simulink model "eq_2khz"  (R2023a)
settings: Solver=VariableStepAuto  StartTime=0.0  StopTime=5.0  RelTol=1e-3
libraries: spspowerguiLib x1
settings Model: Creator=若陈不生病  LastModifiedBy=86198

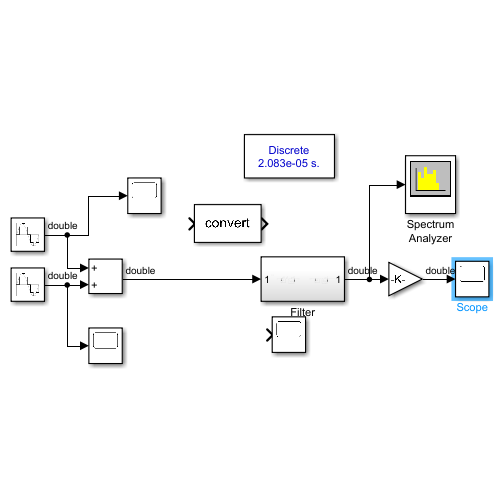
[thumbnail: Simulink's stored preview of the top-level diagram]
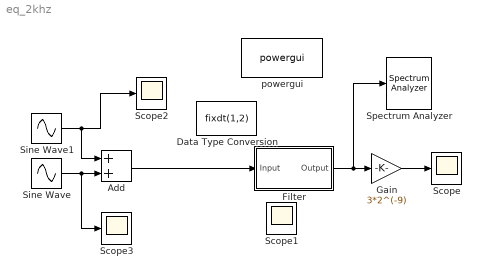
== system eq_2khz ==
  Add : Sum
  Data Type Conversion : DataTypeConversion  OutMin=[-1.1/1.5]  OutMax=[1.1/1.5]  OutDataTypeStr=fixdt(1,2)  SaturateOnIntegerOverflow=off  RndMeth=Floor
  Filter : Subsystem  Tag=FilterWizardSubSystem
      settings: ErrorFcn=dspFilterRealizedInBasicElemsAlgLoopErrFcnCallback
  Gain : Gain  Gain=3*2^(-9)
  Scope{,1..3} (4 alike) : Scope
  Sine Wave : Sin  Frequency=2*pi*200  SampleTime=1/48000
  Sine Wave1 : Sin  Frequency=2*pi*2000  SampleTime=1/48000
  Spectrum Analyzer : SpectrumAnalyzer  WindowPosition=[320.000000,230.000000,800.000000,500.000000,]  Visible=on  ScopeFrameLocation=window  YLimits=[-201.08223669,103.16468539]  ColorLimits=[-20 80]  DefaultConfigurationName=spbscopes.SpectrumAnalyzerBlockCfg  IsFrequencyInputMode=0  FrequencyVectorPort=0  FrequencyVectorFromPort=0  FrequencyInputRBWPort=0  FrequencyInputRBWFromPort=0
  powergui : spspowerguiLib/powergui  Priority=1  SimulationMode=Discrete  SampleTime=1/48000  frequency=60  Iterations=50  frequencyindice=60  Pbase=100e6  ErrMax=1e-4  UnitsV=kV  UnitsW=MW  buscounter=0  FunctionMessages=off  echomessages=off  EnableUseOfTLC=off  CurrentSourceSwitches=off  DisableSnubberDevices=off  DisableRonSwitches=off  DisableVfSwitches=off  DisplayEquations=off  AutomaticDiscreteSolvers=off  SolverType=Tustin/Backward Euler (TBE)  Interpol=off  ExternalGateDelay=off  methode=off  Ts=100  x0status=blocks  SPID=on  SwTol=0  HookPort=off  NonlinearTolerance=1e-4  nMaxIteration=100  ContinueOnMaxIteration=off  RestoreLinks=warning  ResistiveCurrentMeasurement=off  Frange=[0:2:500]  Ylog=off  Xlog=on  ShowGrid=off  save=off  variable=ZData  structure=0  ZoomFFT=off  StartTime=0.0  cycles=1  DisplayStyle=1  fundamental=60  FreqAxis=off  MaxFrequency=1000  frequencyindicesteady=1  RmsSteady=1  display=off
  wires:
  Sine Wave/1 -> Add/2, Scope3/1
  Gain/1 -> Scope/1
  Filter/1(Output) -> Spectrum Analyzer/1, Gain/1
  Sine Wave1/1 -> Scope2/1, Add/1
  Add/1 -> Filter/1(Input)

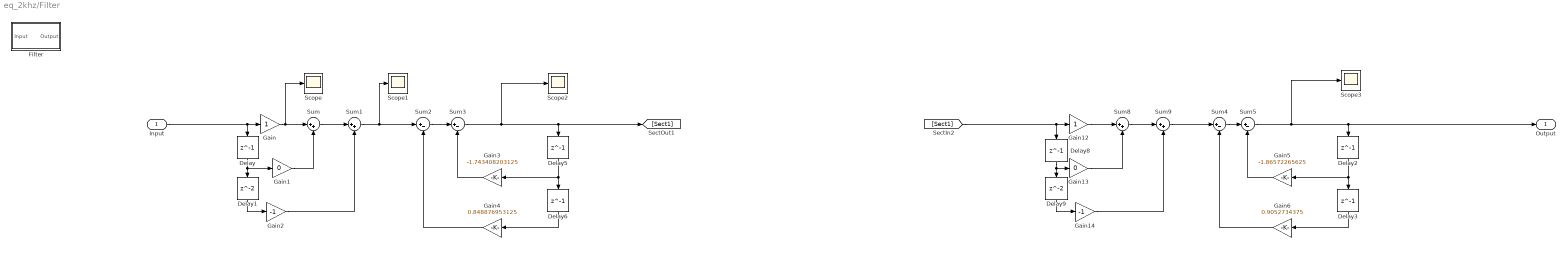
== system eq_2khz/Filter ==
  Input : Inport
  Delay{,2..3,5..6,8} (6 alike) : Delay  DelayLength=1
  Delay1 : Delay
  Delay9 : Delay
  Filter : Subsystem  Tag=FilterWizardSubSystem
      settings: ErrorFcn=dspFilterRealizedInBasicElemsAlgLoopErrFcnCallback
  Gain : Gain
  Gain1 : Gain  Gain=0
  Gain12 : Gain
  Gain13 : Gain  Gain=0
  Gain14 : Gain  Gain=-1
  Gain2 : Gain  Gain=-1
  Gain3 : Gain  Gain=-1.743408203125
  Gain4 : Gain  Gain=0.848876953125
  Gain5 : Gain  Gain=-1.86572265625
  Gain6 : Gain  Gain=0.9052734375
  Scope{,1..3} (4 alike) : Scope
  Sum{,1,8..9} (4 alike) : Sum  Inputs=|++
  Sum{2..5} (4 alike) : Sum  Inputs=|+-
  Output : Outport
  wires:
  Gain13/1 -> Sum8/2
  Delay8/1 -> Delay9/1, Gain13/1
  Gain12/1 -> Sum8/1
  Gain14/1 -> Sum9/2
  Delay9/1 -> Gain14/1
  Sum8/1 -> Sum9/1
  [Sect1] -> Delay8/1, Gain12/1
  Delay6/1 -> Gain4/1
  Delay5/1 -> Delay6/1, Gain3/1
  Gain1/1 -> Sum/2
  Delay/1 -> Delay1/1, Gain1/1
  Gain/1 -> Scope/1, Sum/1
  Gain2/1 -> Sum1/2
  Sum1/1 -> Scope1/1, Sum2/1
  Delay1/1 -> Gain2/1
  Sum/1 -> Sum1/1
  Input/1 -> Gain/1, Delay/1
  Sum2/1 -> Sum3/1
  Gain3/1 -> Sum3/2
  Gain4/1 -> Sum2/2
  Sum3/1 -> Scope2/1, [Sect1], Delay5/1
  Gain6/1 -> Sum4/2
  Sum4/1 -> Sum5/1
  Delay3/1 -> Gain6/1
  Delay2/1 -> Delay3/1, Gain5/1
  Gain5/1 -> Sum5/2
  Sum5/1 -> Scope3/1, Output/1, Delay2/1
  Sum9/1 -> Sum4/1

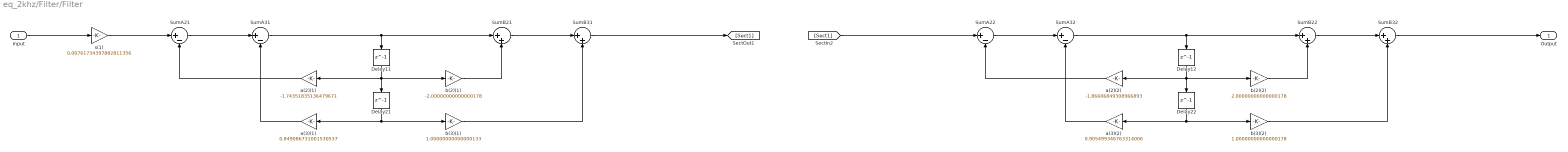
== system eq_2khz/Filter/Filter ==
  Input : Inport
  Delay{11..12,21..22} (4 alike) : Delay  DelayLength=1  InitialCondition=0
  SumA{21..22,31..32} (4 alike) : Sum  Inputs=|+-  RndMeth=Nearest  SaturateOnIntegerOverflow=on  OutDataTypeStr=Inherit: Same as first input
  SumB{21..22,31..32} (4 alike) : Sum  Inputs=|++  RndMeth=Nearest  SaturateOnIntegerOverflow=on  OutDataTypeStr=Inherit: Same as first input
  a(2)(1) : Gain  Gain=-1.74351835136479671  ParamDataTypeStr=double  RndMeth=Nearest  SaturateOnIntegerOverflow=on  OutDataTypeStr=Inherit: Same as input
  a(2)(2) : Gain  Gain=-1.86606849308966893  ParamDataTypeStr=double  RndMeth=Nearest  SaturateOnIntegerOverflow=on  OutDataTypeStr=Inherit: Same as input
  a(3)(1) : Gain  Gain=0.849086731001530537  ParamDataTypeStr=double  RndMeth=Nearest  SaturateOnIntegerOverflow=on  OutDataTypeStr=Inherit: Same as input
  a(3)(2) : Gain  Gain=0.905499346763314006  ParamDataTypeStr=double  RndMeth=Nearest  SaturateOnIntegerOverflow=on  OutDataTypeStr=Inherit: Same as input
  b(2)(1) : Gain  Gain=-2.00000000000000178  ParamDataTypeStr=double  RndMeth=Nearest  SaturateOnIntegerOverflow=on  OutDataTypeStr=Inherit: Same as input
  b(2)(2) : Gain  Gain=2.00000000000000178  ParamDataTypeStr=double  RndMeth=Nearest  SaturateOnIntegerOverflow=on  OutDataTypeStr=Inherit: Same as input
  b(3)(1) : Gain  Gain=1.00000000000000133  ParamDataTypeStr=double  RndMeth=Nearest  SaturateOnIntegerOverflow=on  OutDataTypeStr=Inherit: Same as input
  b(3)(2) : Gain  Gain=1.00000000000000178  ParamDataTypeStr=double  RndMeth=Nearest  SaturateOnIntegerOverflow=on  OutDataTypeStr=Inherit: Same as input
  s(1) : Gain  Gain=0.00761734397882811356  ParamDataTypeStr=double  RndMeth=Nearest  SaturateOnIntegerOverflow=on  OutDataTypeStr=Inherit: Same as input
  Output : Outport
  wires:
  Input/1 -> s(1)/1
  s(1)/1 -> SumA21/1
  SumA21/1 -> SumA31/1
  SumA31/1 -> SumB21/1, Delay11/1
  SumB21/1 -> SumB31/1
  SumB31/1 -> [Sect1]
  a(2)(1)/1 -> SumA21/2
  Delay11/1 -> a(2)(1)/1, b(2)(1)/1, Delay21/1
  b(2)(1)/1 -> SumB21/2
  a(3)(1)/1 -> SumA31/2
  Delay21/1 -> a(3)(1)/1, b(3)(1)/1
  b(3)(1)/1 -> SumB31/2
  [Sect1] -> SumA22/1
  SumA22/1 -> SumA32/1
  SumA32/1 -> SumB22/1, Delay12/1
  SumB22/1 -> SumB32/1
  SumB32/1 -> Output/1
  a(2)(2)/1 -> SumA22/2
  Delay12/1 -> a(2)(2)/1, b(2)(2)/1, Delay22/1
  b(2)(2)/1 -> SumB22/2
  a(3)(2)/1 -> SumA32/2
  Delay22/1 -> a(3)(2)/1, b(3)(2)/1
  b(3)(2)/1 -> SumB32/2
